simulink model "VisionModel"  (Simulink 7.6)
settings: Solver=FixedStepDiscrete  StartTime=0.0  StopTime=0  RelTol=1e-3
values from neighbouring files (symbols this model uses):
  Scale_Down_B = 1    [VisionConstants.m]
  Scale_Down_G = 1    [VisionConstants.m]
  Scale_Down_H = 1    [VisionConstants.m]
  Scale_Down_R = 1    [VisionConstants.m]
  Scale_Down_S = 1    [VisionConstants.m]
  Scale_Down_V = 5    [VisionConstants.m]
  Scale_Forward_B = 1    [VisionConstants.m]
  Scale_Forward_G = 1    [VisionConstants.m]
  Scale_Forward_H = .8    (= 0.8)    [VisionConstants.m]
  Scale_Forward_R = 1    [VisionConstants.m]
  Scale_Forward_S = 1    [VisionConstants.m]
  Scale_Forward_V = 2    [VisionConstants.m]
undefined symbols (not defined in the file or in its folder): Rec, SDTV
libraries: vipconversions x4
settings Model: Creator=Administrator  LastModifiedBy=auvt
settings RTWCC: TargetLang=C++

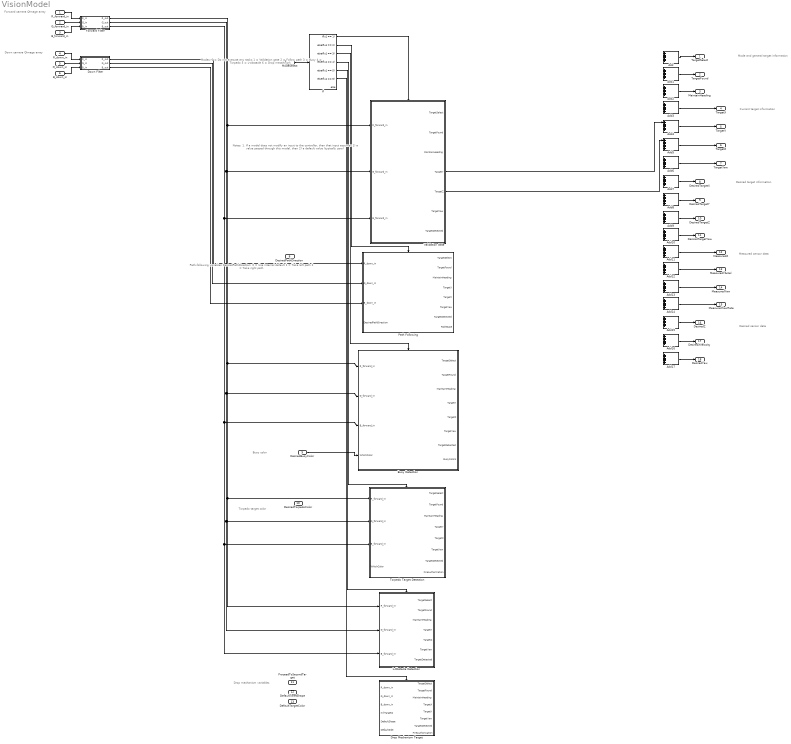
== system VisionModel ==
  note: Current target information
  note: Desired target information
  note: Measured sensor data
  note: Mode and general target information
  note: Desired sensor data
  note: Forward camera QImage array
  note: Modes:
      | 0 = Do not execute any tasks
      | 1 = Validation gate
      | 2 = Follow path
      | 3 = Buoy
      | 4 = Torpedo
      | 5 = L-obstacle
      | 6 = Drop mecahnism
  note: Path-following variables
      | DesiredPathDirection:
      | 0 = Use internal default
      | 1 = Take left path
      | 2 = Take right path
  note: Buoy color
  note: Torpedo target color
  note: Drop mechanism variables
  note: Down camera QImage array
  note: Notes:
      | 1. If a model does not modify an input to the controller,
      | then that input assumes 1) a value passed through this
      | model, then 2) a default value (typically zero)
  R_forward_in : Inport  PortDimensions=Forward_Camera_Dimensions
  G_forward_in : Inport  Port=2  PortDimensions=Forward_Camera_Dimensions
  B_forward_in : Inport  Port=3  PortDimensions=Forward_Camera_Dimensions
  R_down_in : Inport  Port=4  PortDimensions=Down_Camera_Dimensions
  G_down_in : Inport  Port=5  PortDimensions=Down_Camera_Dimensions
  B_down_in : Inport  Port=6  PortDimensions=Down_Camera_Dimensions
  ModeSelect : Inport  Port=7
  DesiredPathDirection : Inport  Port=8
  DesiredBuoyColor : Inport  Port=9
  DesiredTorpedoColor : Inport  Port=10
  ProceedToSecondTarget : Inport  Port=11
  DefaultTaretShape : Inport  Port=12
  DefaultTargetColor : Inport  Port=13
  Add{,1..17} (18 alike) : Sum  Inputs=++++++
  Buoy Detection : Subsystem  TreatAsAtomicUnit=on
  Down Filter : Subsystem
  Drop Mechanism Target : Subsystem  TreatAsAtomicUnit=on
  Forward Filter : Subsystem
  If : If  IfExpression=u1 == 1  ElseIfExpressions=u1 == 2, u1 == 3, u1 == 4, u1 == 5, u1 == 6
  L-Obstacle Detection : Subsystem  TreatAsAtomicUnit=on
  Path Following : Subsystem  TreatAsAtomicUnit=on
  Torpedo Target Detection : Subsystem  TreatAsAtomicUnit=on
  Validation Gate : Subsystem  TreatAsAtomicUnit=on
  TargetSelect : Outport  OutDataTypeStr=double
  TargetFound : Outport  Port=2  OutDataTypeStr=double
  MaintainHeading : Outport  Port=3  OutDataTypeStr=double
  TargetX : Outport  Port=4  OutDataTypeStr=double
  TargetY : Outport  Port=5  OutDataTypeStr=double
  TargetZ : Outport  Port=6  OutDataTypeStr=double
  TargetYaw : Outport  Port=7  OutDataTypeStr=double
  DesiredTargetX : Outport  Port=8  OutDataTypeStr=double
  DesiredTargetY : Outport  Port=9  OutDataTypeStr=double
  DesiredTargetZ : Outport  Port=10  OutDataTypeStr=double
  DesiredTargetYaw : Outport  Port=11  OutDataTypeStr=double
  MeasuredZ : Outport  Port=12  OutDataTypeStr=double
  MeasuredYAccel : Outport  Port=13  OutDataTypeStr=double
  MeasuredYaw : Outport  Port=14  OutDataTypeStr=double
  MeasuredYawRate : Outport  Port=15  OutDataTypeStr=double
  DesiredZ : Outport  Port=16  OutDataTypeStr=double
  DesiredXVelocity : Outport  Port=17  OutDataTypeStr=double
  DesiredYaw : Outport  Port=18  OutDataTypeStr=double
  wires:
  ModeSelect/1 -> If/1
  If/2 -> Path Following/Action
  If/3 -> Buoy Detection/Action
  If/1 -> Validation Gate/Action
  If/4 -> Torpedo Target Detection/Action
  If/5 -> L-Obstacle Detection/Action
  If/6 -> Drop Mechanism Target/Action
  DesiredBuoyColor/1 -> Buoy Detection/4(WhichColor)
  Down Filter/1(R_out) -> Path Following/1(R_down_in)
  Down Filter/2(G_out) -> Path Following/2(G_down_in)
  Down Filter/3(B_out) -> Path Following/3(B_down_in)
  Add/1 -> TargetSelect/1
  Add1/1 -> TargetFound/1
  Add2/1 -> MaintainHeading/1
  Add3/1 -> TargetX/1
  Add4/1 -> TargetY/1
  Add5/1 -> TargetZ/1
  Add6/1 -> TargetYaw/1
  Add7/1 -> DesiredTargetX/1
  Add8/1 -> DesiredTargetY/1
  Add9/1 -> DesiredTargetZ/1
  Add10/1 -> DesiredTargetYaw/1
  Add11/1 -> MeasuredZ/1
  Add12/1 -> MeasuredYAccel/1
  Add13/1 -> MeasuredYaw/1
  Add14/1 -> MeasuredYawRate/1
  Add15/1 -> DesiredZ/1
  Add16/1 -> DesiredXVelocity/1
  Add17/1 -> DesiredYaw/1
  Forward Filter/2(G_out) -> Validation Gate/2(G_forward_in), Buoy Detection/2(G_forward_in), Torpedo Target Detection/2(G_forward_in), L-Obstacle Detection/2(G_forward_in)
  Forward Filter/3(B_out) -> Validation Gate/3(B_forward_in), Buoy Detection/3(B_forward_in), Torpedo Target Detection/3(B_forward_in), L-Obstacle Detection/3(B_forward_in)
  Forward Filter/1(R_out) -> Validation Gate/1(R_forward_in), Buoy Detection/1(R_forward_in), Torpedo Target Detection/1(R_forward_in), L-Obstacle Detection/1(R_forward_in)
  G_down_in/1 -> Down Filter/2(G_in)
  R_down_in/1 -> Down Filter/1(R_in)
  B_down_in/1 -> Down Filter/3(B_in)
  G_forward_in/1 -> Forward Filter/2(G_in)
  R_forward_in/1 -> Forward Filter/1(R_in)
  B_forward_in/1 -> Forward Filter/3(B_in)
  Validation Gate/5(TargetZ) -> Add5/1
  Validation Gate/4(TargetY) -> Add4/1

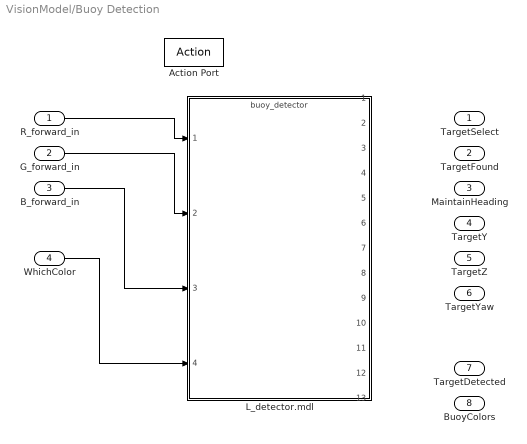
== system VisionModel/Buoy Detection ==
  R_forward_in : Inport
  G_forward_in : Inport  Port=2
  B_forward_in : Inport  Port=3
  WhichColor : Inport  Port=4
  Action Port : ActionPort  ActionType=elseif
  L_detector.mdl : ModelReference  ModelNameDialog=buoy_detector  SimulationMode=Accelerator  ModelReferenceVersion=1.791  CopyOfModelName=buoy_detector
  TargetSelect : Outport  OutDataTypeStr=double
  TargetFound : Outport  Port=2  OutDataTypeStr=double
  MaintainHeading : Outport  Port=3  OutDataTypeStr=double
  TargetY : Outport  Port=4  OutDataTypeStr=double
  TargetZ : Outport  Port=5  OutDataTypeStr=double
  TargetYaw : Outport  Port=6  OutDataTypeStr=double
  TargetDetected : Outport  Port=7  OutDataTypeStr=double
  BuoyColors : Outport  Port=8  OutDataTypeStr=double
  wires:
  R_forward_in/1 -> L_detector.mdl/1
  G_forward_in/1 -> L_detector.mdl/2
  B_forward_in/1 -> L_detector.mdl/3
  WhichColor/1 -> L_detector.mdl/4

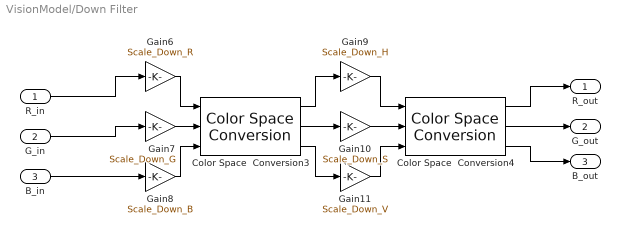
== system VisionModel/Down Filter ==
  R_in : Inport  PortDimensions=Down_Camera_Dimensions
  G_in : Inport  Port=2  PortDimensions=Down_Camera_Dimensions
  B_in : Inport  Port=3  PortDimensions=Down_Camera_Dimensions
  Color Space  Conversion3 : vipconversions/Color Space  Conversion  conversion=Obsolete  conversionActive=R'G'B' to HSV  wp_str=D50  rec=Rec. 601 (SDTV)  sys=1125/60/2:1  imagePorts=Separate color signals
  Color Space  Conversion4 : vipconversions/Color Space  Conversion  conversion=Obsolete  conversionActive=HSV to R'G'B'  wp_str=D50  rec=Rec. 601 (SDTV)  sys=1125/60/2:1  imagePorts=Separate color signals
  Gain10 : Gain  Gain=Scale_Down_S
  Gain11 : Gain  Gain=Scale_Down_V
  Gain6 : Gain  Gain=Scale_Down_R
  Gain7 : Gain  Gain=Scale_Down_G
  Gain8 : Gain  Gain=Scale_Down_B
  Gain9 : Gain  Gain=Scale_Down_H
  R_out : Outport  OutDataTypeStr=double
  G_out : Outport  Port=2  OutDataTypeStr=double
  B_out : Outport  Port=3  OutDataTypeStr=double
  wires:
  Gain6/1 -> Color Space  Conversion3/1
  Gain7/1 -> Color Space  Conversion3/2
  Gain8/1 -> Color Space  Conversion3/3
  Color Space  Conversion3/1 -> Gain9/1
  Color Space  Conversion3/2 -> Gain10/1
  Color Space  Conversion3/3 -> Gain11/1
  Gain9/1 -> Color Space  Conversion4/1
  Gain10/1 -> Color Space  Conversion4/2
  Gain11/1 -> Color Space  Conversion4/3
  R_in/1 -> Gain6/1
  G_in/1 -> Gain7/1
  B_in/1 -> Gain8/1
  Color Space  Conversion4/1 -> R_out/1
  Color Space  Conversion4/2 -> G_out/1
  Color Space  Conversion4/3 -> B_out/1

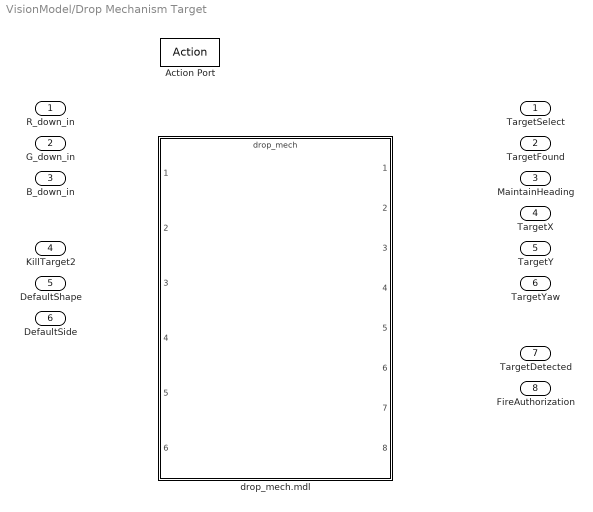
== system VisionModel/Drop Mechanism Target ==
  R_down_in : Inport
  G_down_in : Inport  Port=2
  B_down_in : Inport  Port=3
  KillTarget2 : Inport  Port=4
  DefaultShape : Inport  Port=5
  DefaultSide : Inport  Port=6
  Action Port : ActionPort  ActionType=elseif
  drop_mech.mdl : ModelReference  ModelNameDialog=drop_mech  SimulationMode=Accelerator  ModelReferenceVersion=1.17  CopyOfModelName=drop_mech
  TargetSelect : Outport  OutDataTypeStr=double
  TargetFound : Outport  Port=2  OutDataTypeStr=double
  MaintainHeading : Outport  Port=3  OutDataTypeStr=double
  TargetX : Outport  Port=4  OutDataTypeStr=double
  TargetY : Outport  Port=5  OutDataTypeStr=double
  TargetYaw : Outport  Port=6  OutDataTypeStr=double
  TargetDetected : Outport  Port=7  OutDataTypeStr=double
  FireAuthorization : Outport  Port=8  OutDataTypeStr=double

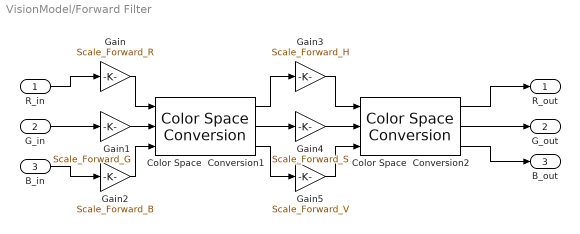
== system VisionModel/Forward Filter ==
  R_in : Inport  PortDimensions=Forward_Camera_Dimensions
  G_in : Inport  Port=2  PortDimensions=Forward_Camera_Dimensions
  B_in : Inport  Port=3  PortDimensions=Forward_Camera_Dimensions
  Color Space  Conversion1 : vipconversions/Color Space  Conversion  conversion=Obsolete  conversionActive=R'G'B' to HSV  wp_str=D50  rec=Rec. 601 (SDTV)  sys=1125/60/2:1  imagePorts=Separate color signals
  Color Space  Conversion2 : vipconversions/Color Space  Conversion  conversion=Obsolete  conversionActive=HSV to R'G'B'  wp_str=D50  rec=Rec. 601 (SDTV)  sys=1125/60/2:1  imagePorts=Separate color signals
  Gain : Gain  Gain=Scale_Forward_R
  Gain1 : Gain  Gain=Scale_Forward_G
  Gain2 : Gain  Gain=Scale_Forward_B
  Gain3 : Gain  Gain=Scale_Forward_H
  Gain4 : Gain  Gain=Scale_Forward_S
  Gain5 : Gain  Gain=Scale_Forward_V
  R_out : Outport  OutDataTypeStr=double
  G_out : Outport  Port=2  OutDataTypeStr=double
  B_out : Outport  Port=3  OutDataTypeStr=double
  wires:
  R_in/1 -> Gain/1
  G_in/1 -> Gain1/1
  B_in/1 -> Gain2/1
  Gain/1 -> Color Space  Conversion1/1
  Gain1/1 -> Color Space  Conversion1/2
  Gain2/1 -> Color Space  Conversion1/3
  Color Space  Conversion1/1 -> Gain3/1
  Color Space  Conversion1/2 -> Gain4/1
  Color Space  Conversion1/3 -> Gain5/1
  Gain3/1 -> Color Space  Conversion2/1
  Gain4/1 -> Color Space  Conversion2/2
  Gain5/1 -> Color Space  Conversion2/3
  Color Space  Conversion2/1 -> R_out/1
  Color Space  Conversion2/2 -> G_out/1
  Color Space  Conversion2/3 -> B_out/1

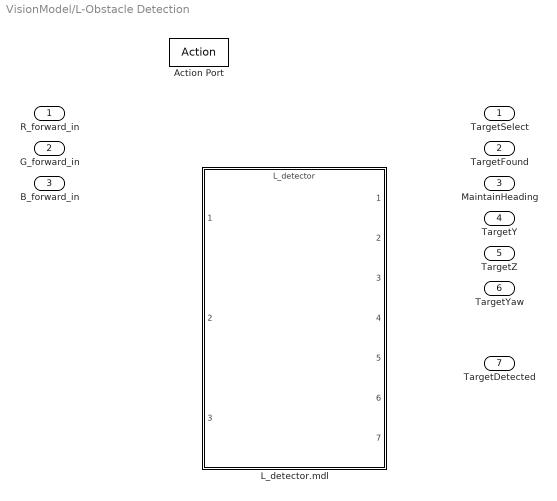
== system VisionModel/L-Obstacle Detection ==
  R_forward_in : Inport
  G_forward_in : Inport  Port=2
  B_forward_in : Inport  Port=3
  Action Port : ActionPort  ActionType=elseif
  L_detector.mdl : ModelReference  ModelNameDialog=L_detector  SimulationMode=Accelerator  ModelReferenceVersion=1.145  CopyOfModelName=L_detector
  TargetSelect : Outport  OutDataTypeStr=double
  TargetFound : Outport  Port=2  OutDataTypeStr=double
  MaintainHeading : Outport  Port=3  OutDataTypeStr=double
  TargetY : Outport  Port=4  OutDataTypeStr=double
  TargetZ : Outport  Port=5  OutDataTypeStr=double
  TargetYaw : Outport  Port=6  OutDataTypeStr=double
  TargetDetected : Outport  Port=7  OutDataTypeStr=double

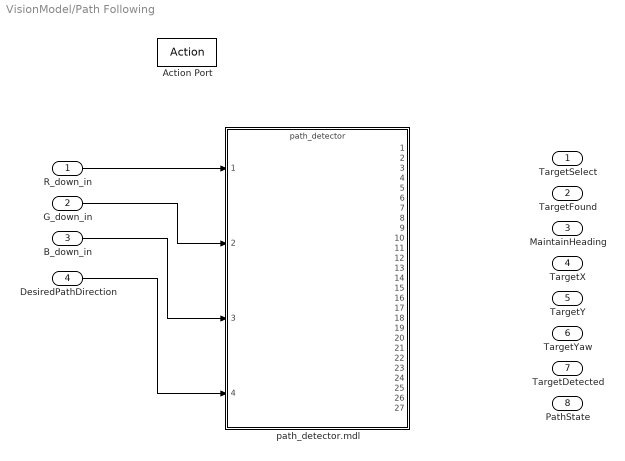
== system VisionModel/Path Following ==
  R_down_in : Inport
  G_down_in : Inport  Port=2
  B_down_in : Inport  Port=3
  DesiredPathDirection : Inport  Port=4
  Action Port : ActionPort  ActionType=elseif
  path_detector.mdl : ModelReference  ModelNameDialog=path_detector  SimulationMode=Accelerator  ModelReferenceVersion=1.303  CopyOfModelName=path_detector
  TargetSelect : Outport  OutDataTypeStr=double
  TargetFound : Outport  Port=2  OutDataTypeStr=double
  MaintainHeading : Outport  Port=3  OutDataTypeStr=double
  TargetX : Outport  Port=4  OutDataTypeStr=double
  TargetY : Outport  Port=5  OutDataTypeStr=double
  TargetYaw : Outport  Port=6  OutDataTypeStr=double
  TargetDetected : Outport  Port=7  OutDataTypeStr=double
  PathState : Outport  Port=8  OutDataTypeStr=double
  wires:
  R_down_in/1 -> path_detector.mdl/1
  G_down_in/1 -> path_detector.mdl/2
  B_down_in/1 -> path_detector.mdl/3
  DesiredPathDirection/1 -> path_detector.mdl/4

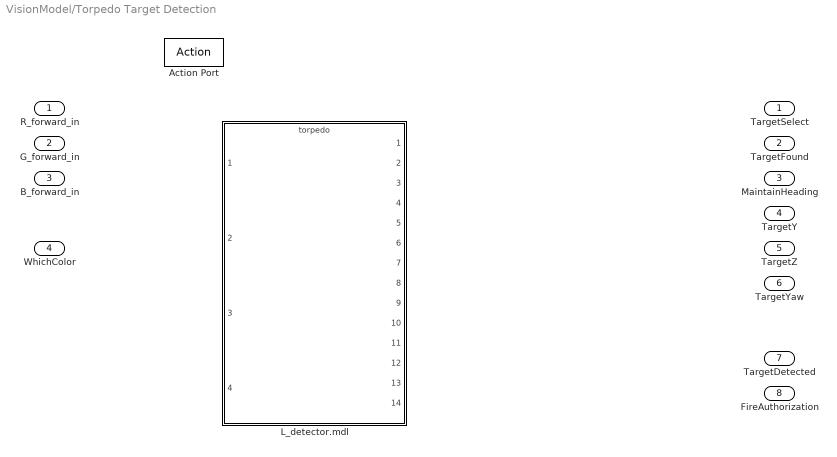
== system VisionModel/Torpedo Target Detection ==
  R_forward_in : Inport
  G_forward_in : Inport  Port=2
  B_forward_in : Inport  Port=3
  WhichColor : Inport  Port=4
  Action Port : ActionPort  ActionType=elseif
  L_detector.mdl : ModelReference  ModelNameDialog=torpedo  SimulationMode=Accelerator  ModelReferenceVersion=1.1048  CopyOfModelName=torpedo
  TargetSelect : Outport  OutDataTypeStr=double
  TargetFound : Outport  Port=2  OutDataTypeStr=double
  MaintainHeading : Outport  Port=3  OutDataTypeStr=double
  TargetY : Outport  Port=4  OutDataTypeStr=double
  TargetZ : Outport  Port=5  OutDataTypeStr=double
  TargetYaw : Outport  Port=6  OutDataTypeStr=double
  TargetDetected : Outport  Port=7  OutDataTypeStr=double
  FireAuthorization : Outport  Port=8  OutDataTypeStr=double

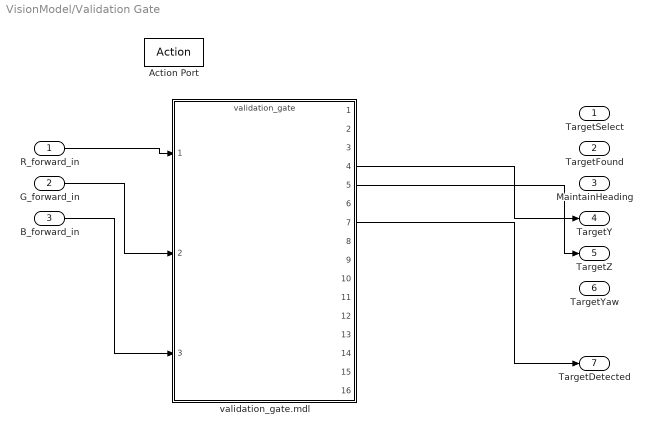
== system VisionModel/Validation Gate ==
  R_forward_in : Inport
  G_forward_in : Inport  Port=2
  B_forward_in : Inport  Port=3
  Action Port : ActionPort  ActionType=then
  validation_gate.mdl : ModelReference  ModelNameDialog=validation_gate  SimulationMode=Accelerator  ModelReferenceVersion=1.1174  CopyOfModelName=validation_gate
  TargetSelect : Outport  OutDataTypeStr=double
  TargetFound : Outport  Port=2  OutDataTypeStr=double
  MaintainHeading : Outport  Port=3  OutDataTypeStr=double
  TargetY : Outport  Port=4  OutDataTypeStr=double
  TargetZ : Outport  Port=5  OutDataTypeStr=double
  TargetYaw : Outport  Port=6  OutDataTypeStr=double
  TargetDetected : Outport  Port=7  OutDataTypeStr=double
  wires:
  R_forward_in/1 -> validation_gate.mdl/1
  G_forward_in/1 -> validation_gate.mdl/2
  B_forward_in/1 -> validation_gate.mdl/3
  validation_gate.mdl/7 -> TargetDetected/1
  validation_gate.mdl/4 -> TargetY/1
  validation_gate.mdl/5 -> TargetZ/1
